simulink model "pipeline_controller"  (Simulink 7.0)
settings: Solver=ode4  StartTime=0.0  StopTime=500  RelTol=1e-3
values from neighbouring files (symbols this model uses):
  bottom = u(7)    [camsim.m]    (also in camsim2.m = u(13); camsim3.m = u(13); initauv.m = 4; wp.m = 10)
undefined symbols (not defined in the file or in its folder): cam_reg
libraries: fordypningsprosjekt x4
settings Model: Creator=anderga  LastModifiedBy=anderga

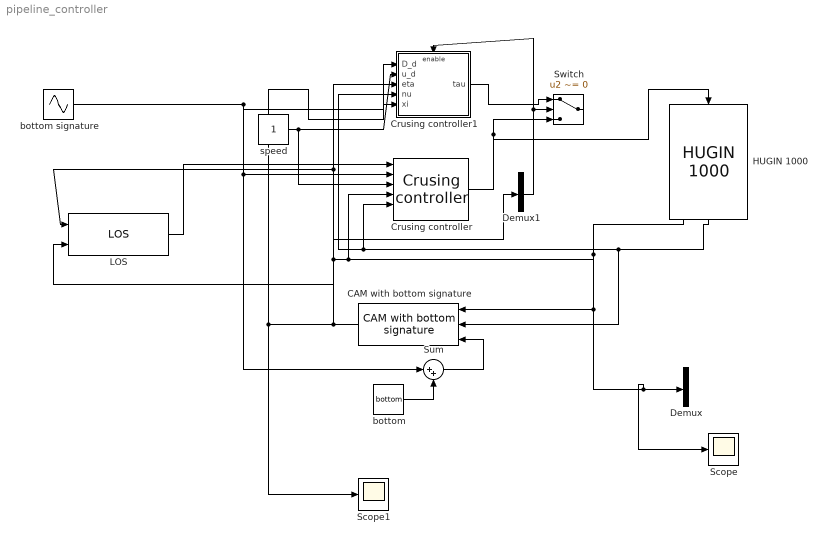
== system pipeline_controller ==
  CAM with bottom signature : fordypningsprosjekt/CAM with bottom signature  Orientation=left  SystemSampleTime=-1  bottom=10
      link override MATLAB Fcn: MATLABFcn=camsim2
  Crusing controller : fordypningsprosjekt/Crusing controller  SystemSampleTime=-1  Kp_u=10  Ki_u=2  Kp_c=100  Kd_c=10  Kp_d=5  Kp2_d=2  Kd_d=4
  Crusing controller1 : Subsystem  AncestorBlock=fordypningsprosjekt/Crusing controller  mask{Kp_u=10, Ki_u=2, Kp_c=100, Kd_c=10, Kp_d=5, Kp2_d=2, Kd_d=4}
      mask prompts: Kp_u "Kp Speed controller"; Ki_u "Ki Speed Controller"; Kp_c "Kp Course Controller"; Kd_c "Kd Course Controller"; Kp_d "Kp1 Depth Controller"; Kp2_d "Kp2 Depth controller"; Kd_d "Kd Depth Controller"
  Demux : Demux  Outputs=6
  Demux1 : Demux  Outputs=6
  HUGIN 1000 : fordypningsprosjekt/HUGIN 1000  Orientation=down  SystemSampleTime=-1  eta_0=[0 0 0 0 0 0]  nu_0=[0 0 0 0 0 0]  c_on_off=on  beta_c=-45  V_c=0.3
  LOS : fordypningsprosjekt/LOS  SystemSampleTime=-1
  Scope : Scope
  Scope1 : Scope
  Sum : Sum  Inputs=|++  OutDataType=sfix(16)  OutScaling=2^0
  Switch : Switch  Criteria=u2 ~= 0  OutDataType=sfix(16)  OutScaling=2^0
  bottom : Constant  Value=bottom  OutDataType=sfix(16)  OutScaling=2^0
  bottom signature : Sin  Amplitude=6  Bias=50  Frequency=0.01  SampleTime=0
  speed : Constant  OutDataType=sfix(16)  OutScaling=2^0
  wires:
  HUGIN 1000/1 -> CAM with bottom signature/1, Demux/1, Scope/1, Crusing controller1/3(eta), LOS/1, LOS/2, Crusing controller/4
  HUGIN 1000/2 -> CAM with bottom signature/2, Crusing controller1/4(nu), Crusing controller/5
  bottom signature/1 -> Crusing controller1/1(D_d), Sum/1, Crusing controller/2
  bottom/1 -> Sum/2
  Sum/1 -> CAM with bottom signature/3
  speed/1 -> Crusing controller1/2(u_d), Crusing controller/3
  CAM with bottom signature/1 -> Scope1/1, Crusing controller1/5(xi), Demux1/1
  LOS/1 -> Crusing controller/1
  Crusing controller1/1(tau) -> Switch/1
  Crusing controller/1 -> Switch/3, HUGIN 1000/1
  Demux1/4 -> Switch/2, Crusing controller1/Enable

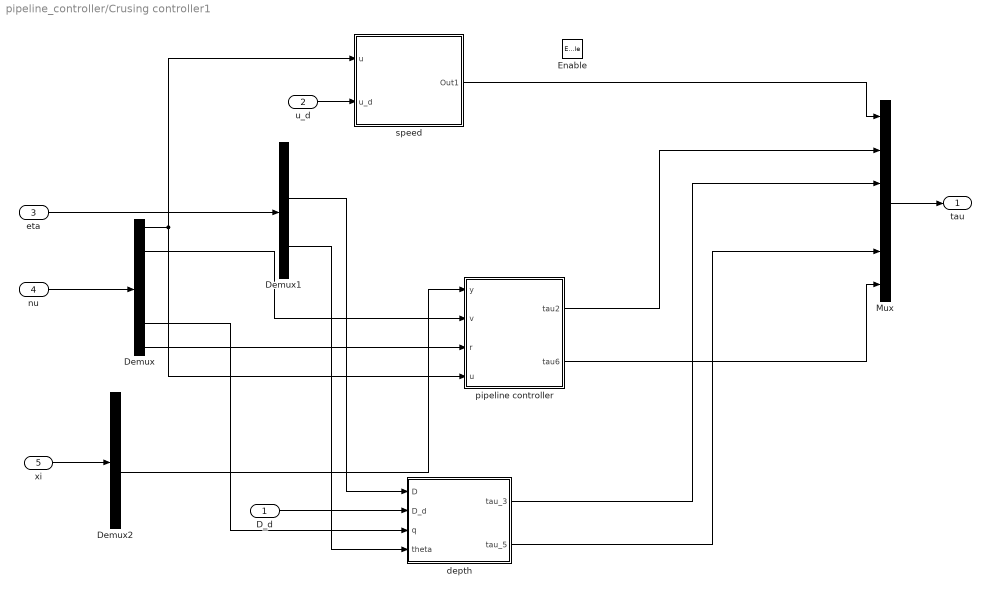
== system pipeline_controller/Crusing controller1 ==
  D_d : Inport  OutDataType=sfix(16)  OutScaling=2^0
  u_d : Inport  Port=2  OutDataType=sfix(16)  OutScaling=2^0
  eta : Inport  Port=3  OutDataType=sfix(16)  OutScaling=2^0
  nu : Inport  Port=4  OutDataType=sfix(16)  OutScaling=2^0
  xi : Inport  Port=5  OutDataType=sfix(16)  OutScaling=2^0
  Enable : EnablePort  StatesWhenEnabling=reset
  Demux : Demux  Outputs=6
  Demux1 : Demux  Outputs=6
  Demux2 : Demux  Outputs=6
  Mux : Mux  Inputs=6
  depth : Subsystem
  pipeline controller : Subsystem
  speed : Subsystem
  tau : Outport  OutDataType=sfix(16)  OutScaling=2^0
  wires:
  depth/2(tau_5) -> Mux/5
  depth/1(tau_3) -> Mux/3
  Demux1/5 -> depth/4(theta)
  Demux/5 -> depth/3(q)
  Demux1/3 -> depth/1(D)
  D_d/1 -> depth/2(D_d)
  Mux/1 -> tau/1
  speed/1(Out1) -> Mux/1
  eta/1 -> Demux1/1
  u_d/1 -> speed/2(u_d)
  Demux/1 -> speed/1(u), pipeline controller/4(u)
  nu/1 -> Demux/1
  Demux/2 -> pipeline controller/2(v)
  Demux/6 -> pipeline controller/3(r)
  pipeline controller/1(tau2) -> Mux/2
  pipeline controller/2(tau6) -> Mux/6
  xi/1 -> Demux2/1
  Demux2/4 -> pipeline controller/1(y)

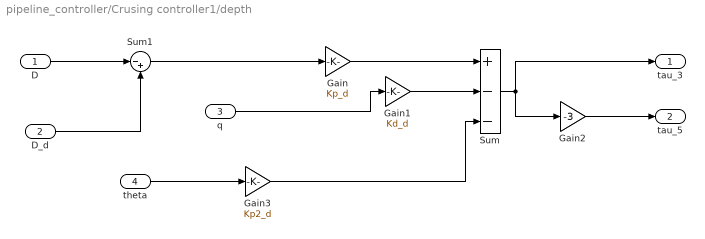
== system pipeline_controller/Crusing controller1/depth ==
  D : Inport  OutDataType=sfix(16)  OutScaling=2^0
  D_d : Inport  Port=2  OutDataType=sfix(16)  OutScaling=2^0
  q : Inport  Port=3  OutDataType=sfix(16)  OutScaling=2^0
  theta : Inport  Port=4  OutDataType=sfix(16)  OutScaling=2^0
  Gain : Gain  Gain=Kp_d  ParameterDataType=sfix(16)  ParameterScaling=2^0  OutDataType=sfix(16)  OutScaling=2^0
  Gain1 : Gain  Gain=Kd_d  ParameterDataType=sfix(16)  ParameterScaling=2^0  OutDataType=sfix(16)  OutScaling=2^0
  Gain2 : Gain  Gain=-3  ParameterDataType=sfix(16)  ParameterScaling=2^0  OutDataType=sfix(16)  OutScaling=2^0
  Gain3 : Gain  Gain=Kp2_d  ParameterDataType=sfix(16)  ParameterScaling=2^0  OutDataType=sfix(16)  OutScaling=2^0
  Sum : Sum  Inputs=+--  OutDataType=sfix(16)  OutScaling=2^0
  Sum1 : Sum  Inputs=|-+  OutDataType=sfix(16)  OutScaling=2^0
  tau_3 : Outport  OutDataType=sfix(16)  OutScaling=2^0
  tau_5 : Outport  Port=2  OutDataType=sfix(16)  OutScaling=2^0
  wires:
  Gain3/1 -> Sum/3
  theta/1 -> Gain3/1
  Sum1/1 -> Gain/1
  Gain1/1 -> Sum/2
  D/1 -> Sum1/1
  D_d/1 -> Sum1/2
  Gain/1 -> Sum/1
  q/1 -> Gain1/1
  Sum/1 -> Gain2/1, tau_3/1
  Gain2/1 -> tau_5/1

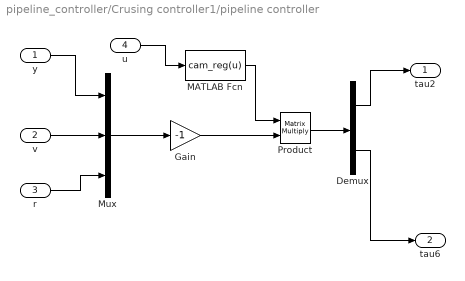
== system pipeline_controller/Crusing controller1/pipeline controller ==
  y : Inport  OutDataType=sfix(16)  OutScaling=2^0
  v : Inport  Port=2  OutDataType=sfix(16)  OutScaling=2^0
  r : Inport  Port=3  OutDataType=sfix(16)  OutScaling=2^0
  u : Inport  Port=4  OutDataType=sfix(16)  OutScaling=2^0
  Demux : Demux  Outputs=2
  Gain : Gain  Gain=-1  ParameterDataType=sfix(16)  ParameterScaling=2^0  OutDataType=sfix(16)  OutScaling=2^0
  MATLAB Fcn : MATLABFcn  MATLABFcn=cam_reg(u)  OutputDimensions=2:3  Output1D=off
  Mux : Mux  Inputs=3
  Product : Product  Multiplication=Matrix(*)  OutDataType=sfix(16)  OutScaling=2^0  RndMeth=Zero
  tau2 : Outport  OutDataType=sfix(16)  OutScaling=2^0
  tau6 : Outport  Port=2  OutDataType=sfix(16)  OutScaling=2^0
  wires:
  y/1 -> Mux/1
  v/1 -> Mux/2
  r/1 -> Mux/3
  u/1 -> MATLAB Fcn/1
  Mux/1 -> Gain/1
  MATLAB Fcn/1 -> Product/1
  Product/1 -> Demux/1
  Demux/1 -> tau2/1
  Demux/2 -> tau6/1
  Gain/1 -> Product/2

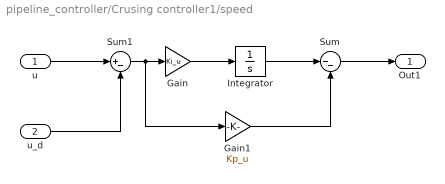
== system pipeline_controller/Crusing controller1/speed ==
  u : Inport  OutDataType=sfix(16)  OutScaling=2^0
  u_d : Inport  Port=2  OutDataType=sfix(16)  OutScaling=2^0
  Gain : Gain  Gain=Ki_u  ParameterDataType=sfix(16)  ParameterScaling=2^0  OutDataType=sfix(16)  OutScaling=2^0
  Gain1 : Gain  Gain=Kp_u  ParameterDataType=sfix(16)  ParameterScaling=2^0  OutDataType=sfix(16)  OutScaling=2^0
  Integrator : Integrator
  Sum : Sum  Inputs=|--  OutDataType=sfix(16)  OutScaling=2^0
  Sum1 : Sum  Inputs=|+-  OutDataType=sfix(16)  OutScaling=2^0
  Out1 : Outport  OutDataType=sfix(16)  OutScaling=2^0
  wires:
  Gain1/1 -> Sum/2
  Gain/1 -> Integrator/1
  Integrator/1 -> Sum/1
  Sum1/1 -> Gain1/1, Gain/1
  u_d/1 -> Sum1/2
  u/1 -> Sum1/1
  Sum/1 -> Out1/1
